simulink model "Simulation"  (R2021a)
settings: Solver=FixedStepAuto  StartTime=0.0  StopTime=20  FixedStep=1e-4  RelTol=1e-3
libraries: simulink_extras x2
settings Model: Creator=libre  LastModifiedBy=libre

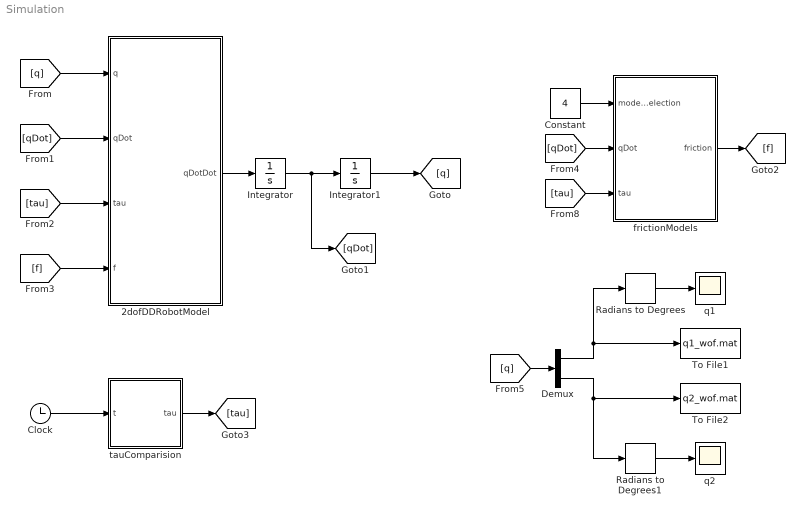
== system Simulation ==
  2dofDDRobotModel : MATLAB Function  TreatAsAtomicUnit=on
  Clock : Clock
  Constant : Constant  Value=4
  Demux : Demux  Outputs=2
  Integrator : Integrator  InitialCondition=[0; 0]
  Integrator1 : Integrator  InitialCondition=[0; 0]
  Radians to Degrees : simulink_extras/Transformations/Radians to Degrees
  Radians to Degrees1 : simulink_extras/Transformations/Radians to Degrees
  To File1 : ToFile  Filename=q1_wof.mat  SaveFormat=Timeseries
  To File2 : ToFile  Filename=q2_wof.mat  SaveFormat=Timeseries
  frictionModels : Subsystem
  q1 : Scope
  q2 : Scope
  tauComparision : MATLAB Function  TreatAsAtomicUnit=on
  wires:
  2dofDDRobotModel/1(qDotDot) -> Integrator/1
  Integrator/1 -> [qDot], Integrator1/1
  Integrator1/1 -> [q]
  [q] -> 2dofDDRobotModel/1(q)
  [qDot] -> 2dofDDRobotModel/2(qDot)
  [f] -> 2dofDDRobotModel/4(f)
  [tau] -> 2dofDDRobotModel/3(tau)
  Constant/1 -> frictionModels/1(model selection)
  [qDot] -> frictionModels/2(qDot)
  frictionModels/1(friction) -> [f]
  tauComparision/1(tau) -> [tau]
  Clock/1 -> tauComparision/1(t)
  [q] -> Demux/1
  Radians to Degrees/1 -> q1/1
  Radians to Degrees1/1 -> q2/1
  [tau] -> frictionModels/3(tau)
  Demux/2 -> Radians to Degrees1/1, To File2/1
  Demux/1 -> To File1/1, Radians to Degrees/1

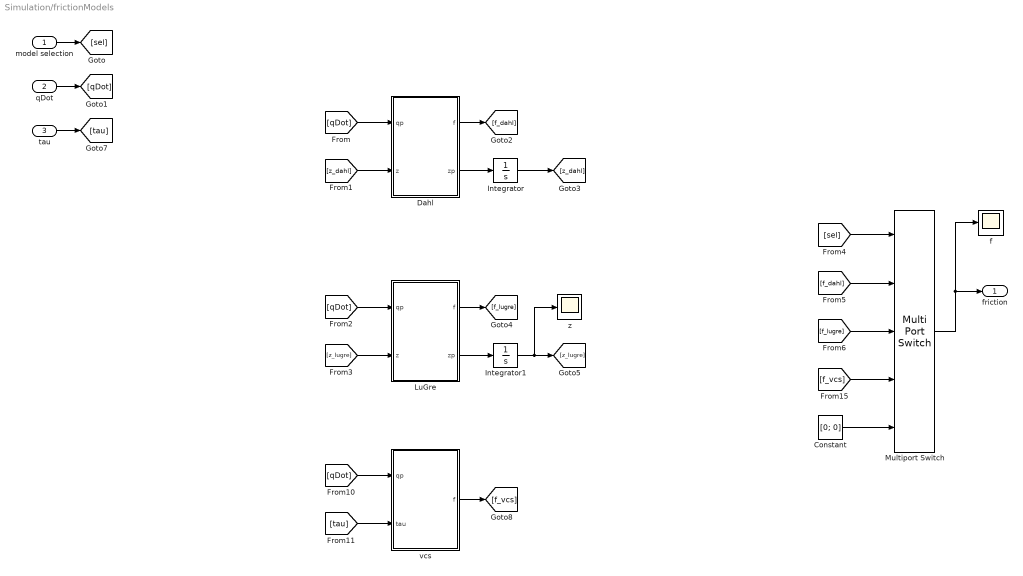
== system Simulation/frictionModels ==
  model selection : Inport
  qDot : Inport  Port=2
  tau : Inport  Port=3
  Constant : Constant  Value=[0; 0]
  Dahl : MATLAB Function  TreatAsAtomicUnit=on
  Integrator : Integrator  InitialCondition=[0; 0]
  Integrator1 : Integrator  InitialCondition=[0; 0]
  LuGre : MATLAB Function  TreatAsAtomicUnit=on
  Multiport Switch : MultiPortSwitch  Inputs=4  DiagnosticForDefault=None
  f : Scope
  vcs : MATLAB Function  TreatAsAtomicUnit=on
  z : Scope
  friction : Outport
  wires:
  model selection/1 -> [sel]
  qDot/1 -> [qDot]
  [qDot] -> Dahl/1(qp)
  [z_dahl] -> Dahl/2(z)
  Dahl/2(zp) -> Integrator/1
  Dahl/1(f) -> [f_dahl]
  Integrator/1 -> [z_dahl]
  LuGre/2(zp) -> Integrator1/1
  [z_lugre] -> LuGre/2(z)
  LuGre/1(f) -> [f_lugre]
  Integrator1/1 -> z/1, [z_lugre]
  [qDot] -> LuGre/1(qp)
  Multiport Switch/1 -> f/1, friction/1
  [sel] -> Multiport Switch/1
  [f_lugre] -> Multiport Switch/3
  [f_dahl] -> Multiport Switch/2
  tau/1 -> [tau]
  vcs/1(f) -> [f_vcs]
  [qDot] -> vcs/1(qp)
  [tau] -> vcs/2(tau)
  [f_vcs] -> Multiport Switch/4
  Constant/1 -> Multiport Switch/5

== matlab function Simulation/frictionModels/Dahl ==
  data: qp input; f output; z input; zp output
function [f,zp] = fcn(qp,z)

sigma_0 = [21418.98; 1013.63];
%%%%%%%%%%%%%%%%%%%%%%%%%%%%%%
sigma_1 = [1404.98; 21.55];
%%%%%%%%%%%%%%%%%%%%%%%%%%%%%%
fc_pos = [12.4401; 1.9181];
fc_neg = [10.9366; 1.7195];
%%%%%%%%%%%%%%%%%%%%%%%%%%%%%%
fs_pos = [10.75; 1.49];
fs_neg = [12.0; 1.45];
%%%%%%%%%%%%%%%%%%%%%%%%%%%%%%
fv_pos = [3.4419; 0.1707];
fv_neg = [2.8016; 0.0839];
%%%%%%%%%%%%%%%%%%%%%%%%%%%%%%
vs_pos = [0.5808*pi/180; 2.678*pi/180];
vs_neg = [0.4301*pi/180; 4.402*pi/180];
%%%%%%%%%%%%%%%%%%%%%%%%%%%%%%
ds_pos = [1.346; 5.025];
ds_neg = [9.971; 4.402];

f = [0; 0];
zp = [0; 0];

for i = 1:2
    if qp(i) > 0 
    f(i) = sigma_0(i)*z(i) + fv_pos(i)*qp(i);
    zp(i) = -sigma_0(i)*abs(qp(i))*z(i)/fc_pos(i) + qp(i);
    else
    f(i) = sigma_0(i)*z(i) + fv_neg(i)*qp(i);
    zp(i) = -sigma_0(i)*abs(qp(i))*z(i)/fc_neg(i) + qp(i);
    end
end

== matlab function Simulation/2dofDDRobotModel ==
  data: q input; qDotDot output; qDot input; tau input; f input
function qDotDot = fcn(q,qDot,tau,f)
g = 9.81;

m11=2.351+0.168*cos(q(2));
m12=0.102+0.084*cos(q(2));
m21=m12;
m22=0.102;

c11=-0.168*sin(q(2))*qDot(2);
c12=-0.084*sin(q(2))*qDot(2);
c21=0.084*sin(q(2))*qDot(1);
c22=0.0;

g1=g*(3.921*sin(q(1))+0.186*sin(q(1) + q(2)));
g2=g*0.186*sin(q(1)+ q(2));

M = [m11 m12; m21 m22];
C = [c11 c12; c21 c22];
g = [g1; g2];

qDotDot = M\(tau - f - C*qDot - g);

== matlab function Simulation/frictionModels/LuGre ==
  data: qp input; f output; z input; zp output
function [f,zp] = fcn(qp,z)

sigma_0 = [21418.98; 1013.63];
%%%%%%%%%%%%%%%%%%%%%%%%%%%%%%
sigma_1 = [1404.98; 21.55];
%%%%%%%%%%%%%%%%%%%%%%%%%%%%%%
fc_pos = [12.4401; 1.9181];
fc_neg = [10.9366; 1.7195];
%%%%%%%%%%%%%%%%%%%%%%%%%%%%%%
fs_pos = [10.75; 1.49];
fs_neg = [12.0; 1.45];
%%%%%%%%%%%%%%%%%%%%%%%%%%%%%%
fv_pos = [3.4419; 0.1707];
fv_neg = [2.8016; 0.0839];
%%%%%%%%%%%%%%%%%%%%%%%%%%%%%%
vs_pos = [0.5808*pi/180; 2.678*pi/180];
vs_neg = [0.4301*pi/180; 4.402*pi/180];
%%%%%%%%%%%%%%%%%%%%%%%%%%%%%%
ds_pos = [1.346; 5.025];
ds_neg = [9.971; 4.402];


f = [0; 0];
zp = [0; 0];

for i = 1:2
    if qp(i) > 0 
    g = fc_pos(i) + (fs_pos(i) - fc_pos(i))*exp(-abs(qp(i)/vs_pos(i))^ds_pos(i));    
    zp(i) = -sigma_0(i)*abs(qp(i))*z(i)/g + qp(i);
    f(i) = sigma_0(i)*z(i) + sigma_1(i)*zp(i) + fv_pos(i)*qp(i);
    else
    g = fc_neg(i) + (fs_neg(i) - fc_neg(i))*exp(-abs(qp(i)/vs_neg(i))^ds_neg(i));
    zp(i) = -sigma_0(i)*abs(qp(i))*z(i)/g + qp(i);
    f(i) = sigma_0(i)*z(i) + sigma_1(i)*zp(i) + fv_neg(i)*qp(i);
    end
end

== matlab function Simulation/tauComparision ==
  data: t input; tau output
function tau = fcn(t)

tau = [20; -2]*sin(2*pi*t*0.1);

== matlab function Simulation/frictionModels/vcs ==
  data: qp input; f output; tau input
function f = fcn(qp,tau)

sigma_0 = [21418.98; 1013.63];
%%%%%%%%%%%%%%%%%%%%%%%%%%%%%%
sigma_1 = [1404.98; 21.55];
%%%%%%%%%%%%%%%%%%%%%%%%%%%%%%
fc_pos = [12.4401; 1.9181];
fc_neg = -[10.9366; 1.7195];
%%%%%%%%%%%%%%%%%%%%%%%%%%%%%%
fs_pos = [10.75; 1.49];
fs_neg = -[12.0; 1.45];
%%%%%%%%%%%%%%%%%%%%%%%%%%%%%%
fv_pos = [3.4419; 0.1707];
fv_neg = [2.8016; 0.0839];
%%%%%%%%%%%%%%%%%%%%%%%%%%%%%%
vs_pos = [0.5808*pi/180; 2.678*pi/180];
vs_neg = [0.4301*pi/180; 4.402*pi/180];
%%%%%%%%%%%%%%%%%%%%%%%%%%%%%%
ds_pos = [1.346; 5.025];
ds_neg = [9.971; 4.402];
f = [0; 0];

for i = 1:2
    if qp(i) > 0 
        f(i) = fc_pos(i) + (fs_pos(i) - fc_pos(i))*exp(-abs(qp(i)/vs_pos(i))^ds_pos(i)) + fv_pos(i)*qp(i);
    elseif qp(i) < 0
        f(i) = fc_neg(i) + (fs_neg(i) - fc_neg(i))*exp(-abs(qp(i)/vs_neg(i))^ds_neg(i)) + fv_neg(i)*qp(i);
    else
        if tau(i) > fs_pos(i)
            f(i) = fs_pos(i);
        elseif tau(i) < fs_neg(i)
            f(i) = fs_neg(i);
        else
           f(i) = tau(i);
        end
    end
end
